simulink model "simulink_file"  (R2020b)
settings: Solver=VariableStepAuto  StartTime=0.0  StopTime=20  FixedStep=0.0005  RelTol=1e-3
settings Model: Creator=Dell Precision  LastModifiedBy=Dell Precision

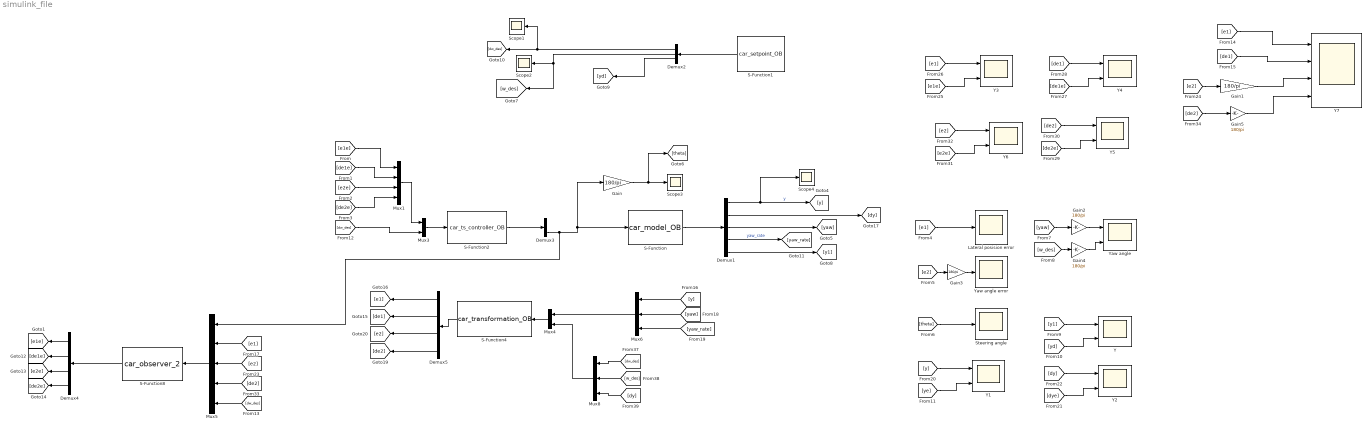
== system simulink_file ==
  Demux1 : Demux  Outputs=5
  Demux2 : Demux  Outputs=3
  Demux3 : Demux  Outputs=2
  Demux4 : Demux
  Demux5 : Demux
  Gain{,1..5} (6 alike) : Gain  Gain=180/pi
  Lateral posision error : Scope
  Mux1 : Mux
  Mux3 : Mux  Inputs=2
  Mux4 : Mux  Inputs=2
  Mux5 : Mux  Inputs=5
  Mux6 : Mux  Inputs=3
  Mux8 : Mux  Inputs=3
  S-Function : S-Function  FunctionName=car_model_OB  SFunctionDeploymentMode=off  EnableBusSupport=off
  S-Function1 : S-Function  FunctionName=car_setpoint_OB  SFunctionDeploymentMode=off  EnableBusSupport=off
  S-Function2 : S-Function  FunctionName=car_ts_controller_OB  SFunctionDeploymentMode=off  EnableBusSupport=off
  S-Function4 : S-Function  FunctionName=car_transformation_OB  SFunctionDeploymentMode=off  EnableBusSupport=off
  S-Function8 : S-Function  FunctionName=car_observer_2  SFunctionDeploymentMode=off  EnableBusSupport=off
  Scope{1..4} (4 alike) : Scope
  Steering angle : Scope
  Y{,1..6} (7 alike) : Scope  NumInputPorts=2
  Y7 : Scope  NumInputPorts=4
  Yaw angle : Scope  NumInputPorts=2
  Yaw angle error : Scope
  wires:
  [e2e] -> Y6/2
  Demux4/1 -> [e1e]
  [de1] -> Y4/1
  [e1] -> Y3/1
  S-Function2/1 -> Demux3/1
  Gain3/1 -> Yaw angle error/1
  [de2e] -> Y5/2
  [e2] -> Gain3/1
  [de1e] -> Y4/2
  [dy] -> Y2/1
  [e2] -> Y6/1
  [de2] -> Y5/1
  Gain4/1 -> Yaw angle/2
  [dye] -> Y2/2
  Gain2/1 -> Yaw angle/1
  Demux5/3 -> [e2]
  [y1] -> Y/1
  [e1] -> Lateral posision error/1
  Demux5/2 -> [de1]
  Mux5/1 -> S-Function8/1
  S-Function1/1 -> Demux2/1
  Demux1/3 -> [yaw]
  Demux1/2 -> [dy]
  [e2e] -> Mux1/3
  Demux1/4 -> [yaw_rate]  "yaw_rate"
  [yaw] -> Gain2/1
  Gain/1 -> [theta], Scope3/1
  Demux2/1 -> Scope1/1, [dw_des]
  Demux1/5 -> [y1]
  [dw_des] -> Mux3/2
  S-Function/1 -> Demux1/1
  [e1e] -> Mux1/1
  [y] -> Mux6/1
  Demux5/1 -> [e1]
  Demux4/4 -> [de2e]
  Mux6/1 -> Mux4/1
  [theta] -> Steering angle/1
  Demux1/1 -> Scope4/1, [y]  "y"
  Demux2/3 -> [yd]
  Mux3/1 -> S-Function2/1
  [de1e] -> Mux1/2
  Mux4/1 -> S-Function4/1
  [yaw] -> Mux6/2
  [ye] -> Y1/2
  [y] -> Y1/1
  [de2e] -> Mux1/4
  Demux4/2 -> [de1e]
  Demux2/2 -> [w_des], Scope2/1
  Mux1/1 -> Mux3/1
  [yaw_rate] -> Mux6/3
  Demux4/3 -> [e2e]
  S-Function4/1 -> Demux5/1
  [e1e] -> Y3/2
  [yd] -> Y/2
  [w_des] -> Gain4/1
  Demux3/2 -> Mux5/1, Gain/1, S-Function/1
  [dw_des] -> Mux8/1
  [w_des] -> Mux8/2
  [dy] -> Mux8/3
  Mux8/1 -> Mux4/2
  Demux5/4 -> [de2]
  [e1] -> Mux5/2
  [e2] -> Mux5/3
  [de2] -> Mux5/4
  [dw_des] -> Mux5/5
  [e1] -> Y7/1
  [de1] -> Y7/2
  [e2] -> Gain1/1
  [de2] -> Gain5/1
  Gain1/1 -> Y7/3
  Gain5/1 -> Y7/4
  S-Function8/1 -> Demux4/1
